simulink model "o1_ar_filter_optimization"  (R2020b)
settings: Solver=FixedStepDiscrete  StartTime=0.0  StopTime=stopTime  RelTol=1e-3
settings Model: Creator=Ross  LastModifiedBy=conno
settings DataIOCC: SaveOutput=off  SaveTime=off  ReturnWorkspaceOutputs=off
settings OptimizationCC: BlockReduction=off  ConditionallyExecuteInputs=off  DefaultParameterBehavior=Inlined
settings DebuggingCC: ReadBeforeWriteMsg=DisableAll  WriteAfterWriteMsg=DisableAll  WriteAfterReadMsg=DisableAll  AlgebraicLoopMsg=error  MultiTaskDSMMsg=none  SingleTaskRateTransMsg=error  PregeneratedLibrarySubsystemCodeDiagnostic=none  ArithmeticOperatorsInVariantConditions=warning
settings HardwareCC: ProdBitPerPointer=32  ProdBitPerSizeT=32  ProdBitPerPtrDiffT=32  ProdLargestAtomicFloat=None  ProdIntDivRoundTo=Undefined  ProdEndianess=Unspecified  ProdWordSize=32  ProdHWDeviceType=ASIC/FPGA->ASIC/FPGA  TargetBitPerPointer=64  TargetBitPerSizeT=64  TargetBitPerPtrDiffT=64  TargetLongLongMode=on  TargetIntDivRoundTo=Zero  TargetEndianess=LittleEndian  TargetWordSize=64  TargetHWDeviceType=Custom Processor->MATLAB Host Computer  ProdEqTarget=off
settings ModelReferenceCC: UpdateModelReferenceTargets=IfOutOfDate
settings SFSimCC: SFSimEcho=off  SimUseLocalCustomCode=off  CustomCodeUndefinedFunction=UseInterfaceOnly
settings RTWCC: RTWUseLocalCustomCode=off

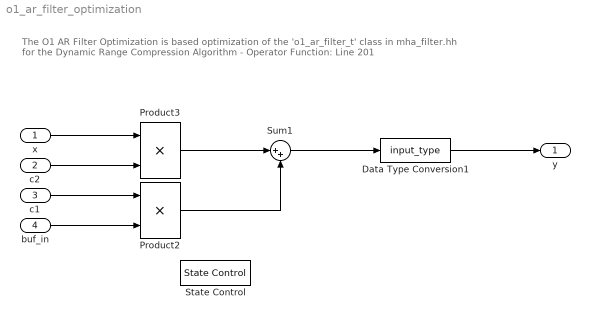
== system o1_ar_filter_optimization ==
  note: The O1 AR Filter Optimization is based optimization of the 'o1_ar_filter_t' class in mha_filter.hh for the Dynamic Range Compression Algorithm
      | - Operator Function: Line 201
  x : Inport  OutDataTypeStr=input_type
  c2 : Inport  Port=2  OutDataTypeStr=ad_coeff_type
  c1 : Inport  Port=3  OutDataTypeStr=ad_coeff_type
  buf_in : Inport  Port=4  OutDataTypeStr=input_type
  Data Type Conversion1 : DataTypeConversion  OutDataTypeStr=input_type  RndMeth=Nearest
  Product2 : Product
  Product3 : Product
  State Control : StateControl  StateControl=Synchronous
  Sum1 : Sum  Inputs=|++  OutDataTypeStr=Inherit: Same as first input
  y : Outport
  wires:
  Product3/1 -> Sum1/1
  Product2/1 -> Sum1/2
  c2/1 -> Product3/2
  buf_in/1 -> Product2/2
  c1/1 -> Product2/1
  x/1 -> Product3/1
  Sum1/1 -> Data Type Conversion1/1
  Data Type Conversion1/1 -> y/1
